simulink model "Noa_Nofusion"  (R2020b)
settings: Solver=FixedStepDiscrete  StartTime=0.0  StopTime=Inf  FixedStep=0.01  RelTol=1e-3
PostLoadFcn:
  | if any(exist('dsrtsu_mdlpostloadfcn', 'file') ~= 0), dsrtsu_mdlpostloadfcn('Execute', bdroot); end
InitFcn:
  | , if any(exist('rtifpga_mdlclblib', 'file') ~= 0), rtifpga_mdlclblib('Init', bdroot); end,
  | , if any(exist('dsmpb_private', 'file') ~= 0), dsmpb_private('dsmpb_mdlclblib', 'Init', bdroot); end,
undefined symbols (not defined in the file or in its folder): ACC_TimeGap_DecSetSwt, ACC_TimeGap_IncSetSwt, AccelPedalPosn, AccelPedalPosnVldty, AccelPedlPosnDiagc, AccPedalOverride, ACU_ShiftInProgress, ADAS_Posn_CurLane, AESSwtReq, ALC_SwtReq, BrkPedalSts, CC_ACC_CANCEL_OFFSwt, CC_ACC_CRUISE_OFFSwt, CC_ACC_DecSetSpd_SetSwt, CC_ACC_IncSetSpd_ResuSwt, CC_ACCSwtErr, CharSpd_ms, CSA_NODE, CURRENT_GEAR, CurrentGearValid, DiscIntNeverNeededParam, DrvDoorSts, DrvSBR, DrvTrqReqOvld, ECMACCInterface, ECMRespACC, ELKSwtReq, EngLimpHomeSts, EngSpd, EngState, EngState_PHEV, EngTrqMaxActSpd, EngTrqMinAct, EPS_DrvInpTrqVal_HighReslolution, EPS_FailSts, EPS_LKATorqOvrlDlvd, EPS_LKATorqOvrlDlvdVld, EPS_LKATrqOvlDlvdSts, EPS_SteerMod, EPS_TrqSnsrSts, EQ4_APPINFO, EQ4_LA_ELEM, EQ4_LA_HDR, EQ4_LAP_ELEM, EQ4_LAP_HDR, EQ4_LH_ELEM, EQ4_LH_HDR, EQ4_LRE_ELEM, EQ4_LRE_HDR, ESS_PedSwtReq, ESS_VehSwtReq, FFogLmpSts_F_Pbox, FLWheelDriveDirection, FLWheelSpd, FrntWiprSwtSts, FrntWshrSwtSts, FRWheelDriveDirection, FRWheelSpd, HazardLmpSwtSts, HCU_AccelPedalPosn_Diag ... (+151)
libraries: simulink x144, dsmpblib x33, canfdmsglib x10
(part 2 of 20)

== system Noa_Nofusion/CAL ==
  Bus Assignment : BusAssignment  AssignedSignals=VehConfigHWA,VehConfigTJA,VehConfigLCK,VehConfigELK,VehConfigACC,VehConfigESS,VehConfigCC,VehConfigLKA,VehConfigLDW,VehConfigLCKIE,VehConfigiACC,VehConfigTSR,VehConfigAES
  Bus Assignment1 : BusAssignment  AssignedSignals=VehConfigADB,VehConfigHMA,VehConfigHMA_laser
  Bus Creator2 : BusCreator  Inputs=2
  Constant1 : Constant  Value=0  OutDataTypeStr=Bus: CAL_AHBC_CONFIG_BUS
  Constant2 : Constant  OutDataTypeStr=uint8
  Constant6 : Constant  Value=0  OutDataTypeStr=Bus: CAL_VSM_CONFIG_BUS
  Constant7 : Constant  OutDataTypeStr=uint8
  IfCALBus : Outport
  wires:
  Constant7/1 -> Bus Assignment/2, Bus Assignment/14, Bus Assignment/13, Bus Assignment/12, Bus Assignment/11, Bus Assignment/10, Bus Assignment/9, Bus Assignment/8, Bus Assignment/7, Bus Assignment/6, Bus Assignment/5, Bus Assignment/4, Bus Assignment/3
  Constant6/1 -> Bus Assignment/1
  Constant2/1 -> Bus Assignment1/4, Bus Assignment1/3, Bus Assignment1/2
  Bus Creator2/1 -> IfCALBus/1  "IfCALBus"
  Bus Assignment1/1 -> Bus Creator2/2  "CAL_AHBC_CONFIG"
  Bus Assignment/1 -> Bus Creator2/1  "CAL_VSM_CONFIG"
  Constant1/1 -> Bus Assignment1/1

== system Noa_Nofusion/CR_RSDS_Input ==
  Bus Assignment3 : BusAssignment  AssignedSignals=Object_ID,Object_DX,Object_DY,Object_VX,Object_VY,Object_AX,Object_Age,Object_MovingState,Object_Fus_Type
  Bus Creator : BusCreator  Inputs=2
  Bus Selector{,1..3} (4 alike) : BusSelector  OutputSignals=ObjAx,ObjMoveSts,ObjFusType,ObjID,ObjAge
  Bus Selector{4..7} (4 alike) : BusSelector  OutputSignals=ObjDx,ObjDy,ObjVx,ObjVy
  CL : MATLAB Function  Commented=on  TreatAsAtomicUnit=on
  CR_L_Bus : Subsystem
  CR_Left_ObjUpdate_b : dsmpblib/Data Inport  Priority=10000
      settings: SourceProductName=dSPACE Model Interface Blockset
  CR_R_Bus : Subsystem
  CR_Right_ObjUpdate_b : dsmpblib/Data Inport  Priority=10000
      settings: SourceProductName=dSPACE Model Interface Blockset
  Constant2 : Constant  Value=24  OutDataTypeStr=uint8
  Constant3 : Constant  Value=0  OutDataTypeStr=Bus: TOS_LC_BUS
  Data Type Conversion : DataTypeConversion
  Detect Change{2..5} (4 alike) : simulink/Logic and Bit Operations/Detect Change  vinit=0  OutDataTypeStr=boolean
  MATLAB Function1 : MATLAB Function  TreatAsAtomicUnit=on
  MATLAB Function2 : MATLAB Function  TreatAsAtomicUnit=on
  Matrix Concatenate{,1..8} (9 alike) : Concatenate  NumInputs=4
  RSDS_L_Bus : Subsystem
  RSDS_Left_ObjUpdate_b : dsmpblib/Data Inport  Priority=10000
      settings: SourceProductName=dSPACE Model Interface Blockset
  RSDS_R_Bus : Subsystem
  RSDS_Right_ObjUpdate_b : dsmpblib/Data Inport  Priority=10000
      settings: SourceProductName=dSPACE Model Interface Blockset
  Unit Delay1 : UnitDelay  Commented=on  SampleTime=-1  HasFrameUpgradeWarning=on
  LC_Obj : Outport  OutDataTypeStr=Bus: TOS_LC_BUS
  LC_ObjIE : Outport  Port=2
  wires:
  Bus Selector5/4 -> Matrix Concatenate5/2  "<ObjVy>"
  [RSDS_L] -> Bus Selector2/1
  CR_Right_ObjUpdate_b/1 -> Detect Change3/1
  Matrix Concatenate8/1 -> [Dx]
  [CR_L] -> Bus Selector4/1
  Bus Selector3/5 -> Matrix Concatenate/4  "<ObjAge>"
  Bus Selector/4 -> Matrix Concatenate1/1  "<ObjID>"
  [RSDS_R] -> Bus Selector3/1
  RSDS_Left_ObjUpdate_b/1 -> Detect Change4/1
  [Vx] -> MATLAB Function2/6(Vx)
  Matrix Concatenate1/1 -> [ID]
  Bus Selector3/4 -> Matrix Concatenate1/4  "<ObjID>"
  Bus Selector1/5 -> Matrix Concatenate/2  "<ObjAge>"
  Bus Selector5/3 -> Matrix Concatenate6/2  "<ObjVx>"
  Bus Selector4/4 -> Matrix Concatenate5/1  "<ObjVy>"
  RSDS_Right_ObjUpdate_b/1 -> Detect Change5/1
  Bus Selector6/1 -> Matrix Concatenate8/3  "<ObjDx>"
  Bus Selector2/4 -> Matrix Concatenate1/3  "<ObjID>"
  Matrix Concatenate2/1 -> [FusType]
  Bus Selector7/2 -> Matrix Concatenate7/4  "<ObjDy>"
  Bus Selector2/2 -> Matrix Concatenate3/3  "<ObjMoveSts>"
  Bus Selector3/2 -> Matrix Concatenate3/4  "<ObjMoveSts>"
  Bus Selector4/1 -> Matrix Concatenate8/1  "<ObjDx>"
  Bus Selector6/2 -> Matrix Concatenate7/3  "<ObjDy>"
  Constant2/1 -> MATLAB Function1/1(ObjNumber)
  Constant3/1 -> Bus Assignment3/1
  [CR_R] -> Bus Selector5/1
  [RSDS_R] -> Bus Selector7/1
  [Dx] -> MATLAB Function2/4(Dx)
  [CR_R] -> Bus Selector1/1
  Bus Selector/5 -> Matrix Concatenate/1  "<ObjAge>"
  [FusType] -> MATLAB Function2/11(FusType)
  Bus Selector1/2 -> Matrix Concatenate3/2  "<ObjMoveSts>"
  CR_Left_ObjUpdate_b/1 -> Detect Change2/1
  Bus Selector6/4 -> Matrix Concatenate5/3  "<ObjVy>"
  Detect Change4/1 -> RSDS_L_Bus/Enable
  Detect Change5/1 -> RSDS_R_Bus/Enable
  Bus Selector/1 -> Matrix Concatenate4/1  "<ObjAx>"
  Detect Change2/1 -> CR_L_Bus/Enable
  Detect Change3/1 -> CR_R_Bus/Enable
  Bus Selector7/3 -> Matrix Concatenate6/4  "<ObjVx>"
  Bus Selector2/5 -> Matrix Concatenate/3  "<ObjAge>"
  Bus Selector3/1 -> Matrix Concatenate4/4  "<ObjAx>"
  Bus Selector7/4 -> Matrix Concatenate5/4  "<ObjVy>"
  [CR_L] -> Bus Selector/1
  MATLAB Function1/2(ObjMatrix) -> MATLAB Function2/2(Matrix)
  Bus Assignment3/1 -> LC_Obj/1
  Bus Selector6/3 -> Matrix Concatenate6/3  "<ObjVx>"
  Bus Selector2/3 -> Matrix Concatenate2/3  "<ObjFusType>"
  Matrix Concatenate3/1 -> [MoveSts]
  Matrix Concatenate7/1 -> [Dy]
  Bus Selector4/2 -> Matrix Concatenate7/1  "<ObjDy>"
  Matrix Concatenate5/1 -> [Vy]
  [Ax] -> MATLAB Function2/8(Ax)
  Bus Selector1/3 -> Matrix Concatenate2/2  "<ObjFusType>"
  Bus Selector2/1 -> Matrix Concatenate4/3  "<ObjAx>"
  [Vy] -> MATLAB Function2/7(Vy)
  Bus Selector3/3 -> Matrix Concatenate2/4  "<ObjFusType>"
  Bus Selector/3 -> Matrix Concatenate2/1  "<ObjFusType>"
  Bus Selector1/1 -> Matrix Concatenate4/2  "<ObjAx>"
  Bus Selector1/4 -> Matrix Concatenate1/2  "<ObjID>"
  Bus Selector5/2 -> Matrix Concatenate7/2  "<ObjDy>"
  [Dx] -> MATLAB Function1/3(ObjDx)
  [RSDS_L] -> Bus Selector6/1
  Bus Selector7/1 -> Matrix Concatenate8/4  "<ObjDx>"
  Bus Selector5/1 -> Matrix Concatenate8/2  "<ObjDx>"
  Bus Selector4/3 -> Matrix Concatenate6/1  "<ObjVx>"
  Bus Selector/2 -> Matrix Concatenate3/1  "<ObjMoveSts>"
  Matrix Concatenate6/1 -> [Vx]
  Matrix Concatenate4/1 -> [Ax]
  [ID] -> MATLAB Function1/2(ObjID)
  Matrix Concatenate/1 -> [Age]
  [Age] -> MATLAB Function2/9(Age)
  [Dy] -> MATLAB Function2/5(Dy)
  [MoveSts] -> MATLAB Function2/10(MoveSts)
  MATLAB Function1/1(ObjPrio) -> MATLAB Function2/1(Prio)
  [ID] -> MATLAB Function2/3(ID)
  RSDS_R_Bus/1(RSDS_R_Obj) -> [RSDS_R]
  RSDS_L_Bus/1(RSDS_L_Obj) -> [RSDS_L]
  CR_L_Bus/1(CR_L_Obj) -> [CR_L]
  CR_R_Bus/1(CR_R_Obj) -> [CR_R]
  CL/9(ObjID) -> Unit Delay1/1
  Unit Delay1/1 -> CL/10(ObjIDK1)
  MATLAB Function2/2(ObjDx) -> Bus Assignment3/3
  MATLAB Function2/1(ObjID) -> Bus Assignment3/2
  MATLAB Function2/3(ObjDy) -> Bus Assignment3/4
  MATLAB Function2/4(ObjVx) -> Bus Assignment3/5
  MATLAB Function2/5(ObjVy) -> Bus Assignment3/6
  MATLAB Function2/6(ObjAx) -> Bus Assignment3/7
  MATLAB Function2/7(ObjAge) -> Data Type Conversion/1
  MATLAB Function2/8(ObjMoveSts) -> Bus Assignment3/9
  MATLAB Function2/9(ObjFusType) -> Bus Assignment3/10
  Data Type Conversion/1 -> Bus Assignment3/8
  [RSDS_L] -> Bus Creator/1  "RL"
  [RSDS_R] -> Bus Creator/2  "RR"
  Bus Creator/1 -> LC_ObjIE/1
